simulink model "w2064930_Yurii_no_PID"  (R2023a)
settings: Solver=VariableStepAuto  StartTime=0.0  StopTime=1000.0  RelTol=1e-3
settings Model: Creator=yurii  LastModifiedBy=w2064930
settings RTWCC: GPUComputeCapability=5.0

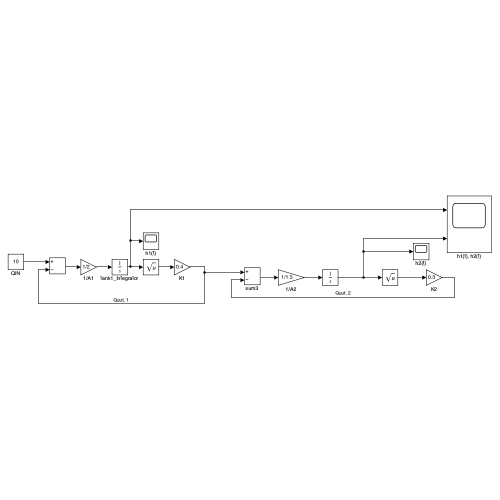
[thumbnail: Simulink's stored preview of the top-level diagram]
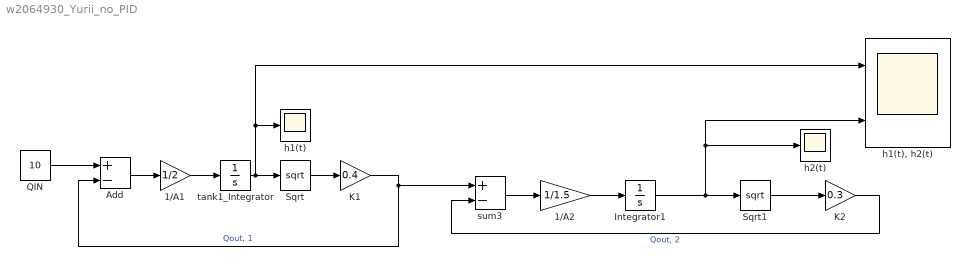
== system w2064930_Yurii_no_PID ==
  1/A1 : Gain  Gain=1/2
  1/A2 : Gain  Gain=1/1.5
  Add : Sum  Inputs=+-
  Integrator1 : Integrator  InitialCondition=0.5
  K1 : Gain  Gain=0.4
  K2 : Gain  Gain=0.3
  QIN : Constant  Value=10
  Sqrt : Sqrt
  Sqrt1 : Sqrt
  h1(t) : Scope
  "h1(t), h2(t)" : Scope  NumInputPorts=2
  h2(t) : Scope
  sum3 : Sum  Inputs=+-
  tank1_Integrator : Integrator  InitialCondition=0.5
  wires:
  K1/1 -> Add/2, sum3/1  "Qout, 1"
  Add/1 -> 1/A1/1
  Sqrt/1 -> K1/1
  1/A1/1 -> tank1_Integrator/1
  tank1_Integrator/1 -> Sqrt/1, "h1(t), h2(t)"/1, h1(t)/1
  Integrator1/1 -> h2(t)/1, "h1(t), h2(t)"/2, Sqrt1/1
  1/A2/1 -> Integrator1/1
  Sqrt1/1 -> K2/1
  sum3/1 -> 1/A2/1
  QIN/1 -> Add/1
  K2/1 -> sum3/2  "Qout, 2"
